simulink model "Exercise12"  (R2016a)
settings: Solver=VariableStepAuto  StartTime=0.0  StopTime=10.0  RelTol=1e-3
values from neighbouring files (symbols this model uses):
  f1 = fs/2-(1*1e3)    (= 499000)    [Exercise1.m]
  f2 = fs/2 + (2*1e3)    (= 502000)    [Exercise1.m]
  f3 = fs+3*1e3    (= 1003000)    [Exercise1.m]
  f4 = fs+7*1e3    (= 1007000)    [Exercise1.m]
  Ts = 1/fs    (= 1e-06)    [Exercise1.m]
undefined symbols (not defined in the file or in its folder): den, num
settings Model: Creator=sergi  LastModifiedBy=sergi

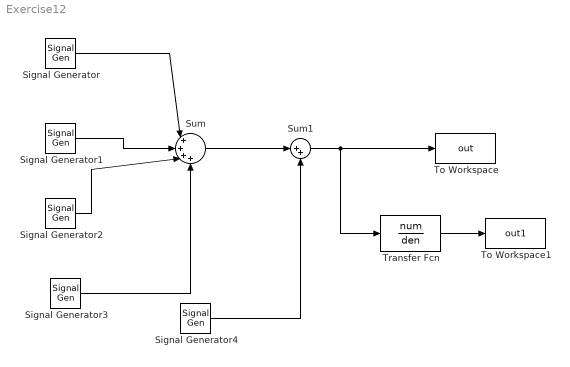
== system Exercise12 ==
  Signal Generator : SignalGenerator  Amplitude=0.1  Frequency=f1
  Signal Generator1 : SignalGenerator  Amplitude=0.01  Frequency=f2
  Signal Generator2 : SignalGenerator  Amplitude=0.1  Frequency=f3
  Signal Generator3 : SignalGenerator  Amplitude=0.01  Frequency=f4
  Signal Generator4 : SignalGenerator  Frequency=10000
  Sum : Sum  Inputs=|++++
  Sum1 : Sum  Inputs=|++
  To Workspace : ToWorkspace  VariableName=out  SampleTime=Ts
      settings: Save2DSignal=2-D array (concatenate along first dimension)
  To Workspace1 : ToWorkspace  VariableName=out1  SampleTime=Ts
      settings: Save2DSignal=2-D array (concatenate along first dimension)
  Transfer Fcn : TransferFcn  Numerator=num  Denominator=den
  wires:
  Signal Generator/1 -> Sum/1
  Signal Generator1/1 -> Sum/2
  Signal Generator2/1 -> Sum/3
  Signal Generator3/1 -> Sum/4
  Sum/1 -> Sum1/1
  Signal Generator4/1 -> Sum1/2
  Sum1/1 -> Transfer Fcn/1, To Workspace/1
  Transfer Fcn/1 -> To Workspace1/1
